simulink library "IOBlock_Library_TTC580"  (R2021a)
settings: Solver=ode45  StartTime=0.0  StopTime=10.0  RelTol=1e-3
PreLoadFcn:
  | addpath(genpath(fileparts(which('IOBlock_Library_TTC580'))));
  | %addpath(genpath(fileparts(which('IOBlock_Library_TTC580.mdl'))))
  | try
  | addpath(genpath([fileparts(which('IOBlock_Library_TTC580')),'\..\DBC_Importer']));
  | addpath(genpath([fileparts(which('IOBlock_Library_TTC580')),'\..\EEPROM_Importer']));
  | addpath(genpath([fileparts(which('IOBlock_Library_TTC580')),'\..\UserDoc']));
  | catch
  | warning('IOBlock_Library_TTC580: add path to DBC_Importer and EEPROM_Importer manually');
  | end
  | try
  | if exist('..\CustomPackage\scripts\OpenAllPackages.m','file')
  |      run('..\CustomPackage\scripts\OpenAllPackages.m'); %always available, ggf. empty
  | end
  | catch
  | warning('A problem occurred opening automatically the CustomPackage. Please open libraries manually');
  | end
  | try
  | set_param(0,'EditorSmartEditingHotParam','off');
  | catch
  | warning('Simlink preferences for ''Edit key parameter when adding new blocks'' needs to be unchecked manually');
  | end
undefined symbols (not defined in the file or in its folder): ADC_Absolute_10V, ADC_Absolute_32V, ADC_Absolute_5V, ADC_BoardTemp, ADC_ChannelInit, ADC_Current, ADC_Get, ADC_K15_, ADC_Ratiometric_10V, ADC_Ratiometric_5V, ADC_Resistive, ADC_SensorSupply, ADC_UBAT, bit_packing, bit_unpacking, CAN_ConfigMsg, compare2error, compare2FET_PROT_REENABLE, crc32_calc_intern, CRC32_EEPROM_Read, CRC32_EEPROM_Write, DIAG_EnterSafestate, DIAG_Status, DIAG_Status_internal, EEPROM_Mirror, EEPROM_Read, EEPROM_Read_OffsetIn, EEPROM_Read_Raw, EEPROM_Write, EEPROM_Write_OffsetIn, EEPROM_Write_Raw, EnterSafestate, FPU_Handler, Get_DI, Get_DI_VarThreshold, Get_K15_, Get_Pulse_Freq_Curr, Get_Pulse_Freq_Volt, Get_WakeUp, GetDateAndTime, IO_ADC_ResetProtection, IO_Blk_Lib_TTC500, IO_CAN_ReadMsg, IO_CAN_WriteMsg, IO_DI_Get, IO_DI_Init, IO_DI_Init_Var, IO_DO_GetCur, IO_DO_GetVoltage, IO_DO_Init, IO_DO_ResetProtection, IO_DO_Set, IO_Driver_GetSerialNumber, IO_Driver_GetVersionOfDriver, IO_Driver_GetVersionOfFPGA, IO_EEPROM_GetStatus, IO_EEPROM_Init, IO_EEPROM_Read_raw, IO_EEPROM_Write, IO_EEPROM_Write_OffsetIn ... (+73)
libraries: simulink x43
(part 15 of 18)

== system IOBlock_Library_TTC580/System  Blocks TTC580 IOlib/Power_Enable ==
  enable : Inport  OutDataTypeStr=boolean  PortDimensions=1
  Data Type Conversion : DataTypeConversion  OutDataTypeStr=uint8
  IO_POWER_Set_POWERSTAGE : Subsystem  LoadFcn=|  mask(IO_POWER_Set_Code){SampleTime=-1, ttlib=IO_Blk_Lib_TTC500, ttDescription=IO_POWER_Set, tt_iolib_version=0.19, pin=IO_INT_POWERSTAGE_ENABLE}
      | try
      | %
      | %Upgrade Information - standard BEGIN
      | new_color = 'blue';
      | new_ver = '0.19';
      | act_ver = get_param(gcb,'tt_iolib_version');
      | if not(strcmp(act_ver,new_ver))
      |     disp(['Upgrade block: ',gcb,char(10),'       Version: ',act_ver,' -> ',new_ver]);
      |     %switch - case for specific upgrade information e.g. additional parameter required 
      |     %Change appearance and version information
      |     set_param(gcb,'ForegroundColor',new_color);
      |     set_param(gcb,'tt_iolib_version',new_ver);
      | end
      | %Upgrade Information - standard END
      | catch
      | %Standard catch section BEGIN 
      | disp(' ');
      | disp('------------------------------------------------------------');
      | disp('An error occurred in a callback of the TTC580-BlockLib.');
      | disp(['Please check the parameters in the mask of ',gcb]);
      | disp('If you do not encounter any violations, then please '); 
      | disp('copy the following lines and report this to support@ttcontrol.com ');
      | disp('<< begin of error message dump >>');
      | disp(['Version of TTC580-BlockLib: ', get_param(gcb,'tt_iolib_version')]);
      | disp(get_param(gcb,'ttDescription'));
      | disp(gcb);
      | x=lasterror;disp(x.message);
      | disp(get_param(gcb,'MaskValues'));
      | disp(version);
      | disp(computer);
      | disp('<< end of error message dump >>');
      | disp('------------------------------------------------------------');
      | disp(' ');
      | %Standard catch section END
      | end
      mask help: Sets a certain mode of the Power IC.
      mask init:
      | %
      settings: CopyFcn=%deleted
      mask Help: web(which('IO_POWER.h'))
      mask TypeOptions pin: IO_INT_POWERSTAGE_ENABLE | IO_SENSOR_SUPPLY_0 | IO_SENSOR_SUPPLY_1 | IO_SENSOR_SUPPLY_2 | IO_INT_SAFETY_SW_0 | IO_INT_SAFETY_SW_1 | IO_INT_SAFETY_SW_2 | IO_K15 | IO_WAKEUP
      mask Callback pin: %
  IO_POWER_Set_SSW0 : Subsystem  LoadFcn=|  mask(IO_POWER_Set_Code){SampleTime=-1, ttlib=IO_Blk_Lib_TTC500, ttDescription=IO_POWER_Set, tt_iolib_version=0.19, pin=IO_INT_SAFETY_SW_0}
      | try
      | %
      | %Upgrade Information - standard BEGIN
      | new_color = 'blue';
      | new_ver = '0.19';
      | act_ver = get_param(gcb,'tt_iolib_version');
      | if not(strcmp(act_ver,new_ver))
      |     disp(['Upgrade block: ',gcb,char(10),'       Version: ',act_ver,' -> ',new_ver]);
      |     %switch - case for specific upgrade information e.g. additional parameter required 
      |     %Change appearance and version information
      |     set_param(gcb,'ForegroundColor',new_color);
      |     set_param(gcb,'tt_iolib_version',new_ver);
      | end
      | %Upgrade Information - standard END
      | catch
      | %Standard catch section BEGIN 
      | disp(' ');
      | disp('------------------------------------------------------------');
      | disp('An error occurred in a callback of the TTC580-BlockLib.');
      | disp(['Please check the parameters in the mask of ',gcb]);
      | disp('If you do not encounter any violations, then please '); 
      | disp('copy the following lines and report this to support@ttcontrol.com ');
      | disp('<< begin of error message dump >>');
      | disp(['Version of TTC580-BlockLib: ', get_param(gcb,'tt_iolib_version')]);
      | disp(get_param(gcb,'ttDescription'));
      | disp(gcb);
      | x=lasterror;disp(x.message);
      | disp(get_param(gcb,'MaskValues'));
      | disp(version);
      | disp(computer);
      | disp('<< end of error message dump >>');
      | disp('------------------------------------------------------------');
      | disp(' ');
      | %Standard catch section END
      | end
      mask help: Sets a certain mode of the Power IC.
      mask init:
      | %
      settings: CopyFcn=%deleted
      mask Help: web(which('IO_POWER.h'))
      mask TypeOptions pin: IO_INT_POWERSTAGE_ENABLE | IO_SENSOR_SUPPLY_0 | IO_SENSOR_SUPPLY_1 | IO_SENSOR_SUPPLY_2 | IO_INT_SAFETY_SW_0 | IO_INT_SAFETY_SW_1 | IO_INT_SAFETY_SW_2 | IO_K15 | IO_WAKEUP
      mask Callback pin: %
  IO_POWER_Set_SSW1 : Subsystem  LoadFcn=|  mask(IO_POWER_Set_Code){SampleTime=-1, ttlib=IO_Blk_Lib_TTC500, ttDescription=IO_POWER_Set, tt_iolib_version=0.19, pin=IO_INT_SAFETY_SW_1}
      | try
      | %
      | %Upgrade Information - standard BEGIN
      | new_color = 'blue';
      | new_ver = '0.19';
      | act_ver = get_param(gcb,'tt_iolib_version');
      | if not(strcmp(act_ver,new_ver))
      |     disp(['Upgrade block: ',gcb,char(10),'       Version: ',act_ver,' -> ',new_ver]);
      |     %switch - case for specific upgrade information e.g. additional parameter required 
      |     %Change appearance and version information
      |     set_param(gcb,'ForegroundColor',new_color);
      |     set_param(gcb,'tt_iolib_version',new_ver);
      | end
      | %Upgrade Information - standard END
      | catch
      | %Standard catch section BEGIN 
      | disp(' ');
      | disp('------------------------------------------------------------');
      | disp('An error occurred in a callback of the TTC580-BlockLib.');
      | disp(['Please check the parameters in the mask of ',gcb]);
      | disp('If you do not encounter any violations, then please '); 
      | disp('copy the following lines and report this to support@ttcontrol.com ');
      | disp('<< begin of error message dump >>');
      | disp(['Version of TTC580-BlockLib: ', get_param(gcb,'tt_iolib_version')]);
      | disp(get_param(gcb,'ttDescription'));
      | disp(gcb);
      | x=lasterror;disp(x.message);
      | disp(get_param(gcb,'MaskValues'));
      | disp(version);
      | disp(computer);
      | disp('<< end of error message dump >>');
      | disp('------------------------------------------------------------');
      | disp(' ');
      | %Standard catch section END
      | end
      mask help: Sets a certain mode of the Power IC.
      mask init:
      | %
      settings: CopyFcn=%deleted
      mask Help: web(which('IO_POWER.h'))
      mask TypeOptions pin: IO_INT_POWERSTAGE_ENABLE | IO_SENSOR_SUPPLY_0 | IO_SENSOR_SUPPLY_1 | IO_SENSOR_SUPPLY_2 | IO_INT_SAFETY_SW_0 | IO_INT_SAFETY_SW_1 | IO_INT_SAFETY_SW_2 | IO_K15 | IO_WAKEUP
      mask Callback pin: %
  IO_POWER_Set_SSW2 : Subsystem  LoadFcn=|  mask(IO_POWER_Set_Code){SampleTime=-1, ttlib=IO_Blk_Lib_TTC500, ttDescription=IO_POWER_Set, tt_iolib_version=0.19, pin=IO_INT_SAFETY_SW_2}
      | try
      | %
      | %Upgrade Information - standard BEGIN
      | new_color = 'blue';
      | new_ver = '0.19';
      | act_ver = get_param(gcb,'tt_iolib_version');
      | if not(strcmp(act_ver,new_ver))
      |     disp(['Upgrade block: ',gcb,char(10),'       Version: ',act_ver,' -> ',new_ver]);
      |     %switch - case for specific upgrade information e.g. additional parameter required 
      |     %Change appearance and version information
      |     set_param(gcb,'ForegroundColor',new_color);
      |     set_param(gcb,'tt_iolib_version',new_ver);
      | end
      | %Upgrade Information - standard END
      | catch
      | %Standard catch section BEGIN 
      | disp(' ');
      | disp('------------------------------------------------------------');
      | disp('An error occurred in a callback of the TTC580-BlockLib.');
      | disp(['Please check the parameters in the mask of ',gcb]);
      | disp('If you do not encounter any violations, then please '); 
      | disp('copy the following lines and report this to support@ttcontrol.com ');
      | disp('<< begin of error message dump >>');
      | disp(['Version of TTC580-BlockLib: ', get_param(gcb,'tt_iolib_version')]);
      | disp(get_param(gcb,'ttDescription'));
      | disp(gcb);
      | x=lasterror;disp(x.message);
      | disp(get_param(gcb,'MaskValues'));
      | disp(version);
      | disp(computer);
      | disp('<< end of error message dump >>');
      | disp('------------------------------------------------------------');
      | disp(' ');
      | %Standard catch section END
      | end
      mask help: Sets a certain mode of the Power IC.
      mask init:
      | %
      settings: CopyFcn=%deleted
      mask Help: web(which('IO_POWER.h'))
      mask TypeOptions pin: IO_INT_POWERSTAGE_ENABLE | IO_SENSOR_SUPPLY_0 | IO_SENSOR_SUPPLY_1 | IO_SENSOR_SUPPLY_2 | IO_INT_SAFETY_SW_0 | IO_INT_SAFETY_SW_1 | IO_INT_SAFETY_SW_2 | IO_K15 | IO_WAKEUP
      mask Callback pin: %
  Terminator_enable{,1..3} (4 alike) : Terminator
  wires:
  enable/1 -> Data Type Conversion/1
  Data Type Conversion/1 -> IO_POWER_Set_POWERSTAGE/1(mode), IO_POWER_Set_SSW0/1(mode), IO_POWER_Set_SSW1/1(mode), IO_POWER_Set_SSW2/1(mode)
  IO_POWER_Set_POWERSTAGE/1(ErrorCode) -> Terminator_enable/1
  IO_POWER_Set_SSW0/1(ErrorCode) -> Terminator_enable1/1
  IO_POWER_Set_SSW1/1(ErrorCode) -> Terminator_enable2/1
  IO_POWER_Set_SSW2/1(ErrorCode) -> Terminator_enable3/1

== system IOBlock_Library_TTC580/System  Blocks TTC580 IOlib/SetDateAndTime ==
  trigger : Inport  OutDataTypeStr=boolean  PortDimensions=1
  seconds : Inport  Port=2  OutDataTypeStr=uint8  PortDimensions=1
  minutes : Inport  Port=3  OutDataTypeStr=uint8  PortDimensions=1
  hours : Inport  Port=4  OutDataTypeStr=uint8  PortDimensions=1
  days : Inport  Port=5  OutDataTypeStr=uint8  PortDimensions=1
  months : Inport  Port=6  OutDataTypeStr=uint8  PortDimensions=1
  years : Inport  Port=7  OutDataTypeStr=uint8  PortDimensions=1
  IO_RTC_GetDateAndTimeStatus : Subsystem  LoadFcn=|  mask(IO_RTC_GetDateAndTimeStatus_Code){SampleTime=-1, ttlib=IO_Blk_Lib_TTC500, ttDescription=IO_RTC_GetDateAndTimeStatus, tt_iolib_version=0.19}
      | try
      | %
      | %Upgrade Information - standard BEGIN
      | new_color = 'blue';
      | new_ver = '0.19';
      | act_ver = get_param(gcb,'tt_iolib_version');
      | if not(strcmp(act_ver,new_ver))
      |     disp(['Upgrade block: ',gcb,char(10),'       Version: ',act_ver,' -> ',new_ver]);
      |     %switch - case for specific upgrade information e.g. additional parameter required 
      |     %Change appearance and version information
      |     set_param(gcb,'ForegroundColor',new_color);
      |     set_param(gcb,'tt_iolib_version',new_ver);
      | end
      | %Upgrade Information - standard END
      | catch
      | %Standard catch section BEGIN 
      | disp(' ');
      | disp('------------------------------------------------------------');
      | disp('An error occurred in a callback of the TTC580-BlockLib.');
      | disp(['Please check the parameters in the mask of ',gcb]);
      | disp('If you do not encounter any violations, then please '); 
      | disp('copy the following lines and report this to support@ttcontrol.com ');
      | disp('<< begin of error message dump >>');
      | disp(['Version of TTC580-BlockLib: ', get_param(gcb,'tt_iolib_version')]);
      | disp(get_param(gcb,'ttDescription'));
      | disp(gcb);
      | x=lasterror;disp(x.message);
      | disp(get_param(gcb,'MaskValues'));
      | disp(version);
      | disp(computer);
      | disp('<< end of error message dump >>');
      | disp('------------------------------------------------------------');
      | disp(' ');
      | %Standard catch section END
      | end
      mask help: Gets the status of the external RTC device.
      mask init:
      | %
      settings: CopyFcn=%deleted
      mask Help: No further help available for this block
  IO_RTC_InitDateAndTime : Subsystem  LoadFcn=|  mask(IO_RTC_InitDateAndTime_Code){SampleTime=-1, ttlib=IO_Blk_Lib_TTC500, ttDescription=IO_RTC_InitDateAndTime, tt_iolib_version=0.19}
      | try
      | %
      | %Upgrade Information - standard BEGIN
      | new_color = 'blue';
      | new_ver = '0.19';
      | act_ver = get_param(gcb,'tt_iolib_version');
      | if not(strcmp(act_ver,new_ver))
      |     disp(['Upgrade block: ',gcb,char(10),'       Version: ',act_ver,' -> ',new_ver]);
      |     %switch - case for specific upgrade information e.g. additional parameter required 
      |     %Change appearance and version information
      |     set_param(gcb,'ForegroundColor',new_color);
      |     set_param(gcb,'tt_iolib_version',new_ver);
      | end
      | %Upgrade Information - standard END
      | catch
      | %Standard catch section BEGIN 
      | disp(' ');
      | disp('------------------------------------------------------------');
      | disp('An error occurred in a callback of the TTC580-BlockLib.');
      | disp(['Please check the parameters in the mask of ',gcb]);
      | disp('If you do not encounter any violations, then please '); 
      | disp('copy the following lines and report this to support@ttcontrol.com ');
      | disp('<< begin of error message dump >>');
      | disp(['Version of TTC580-BlockLib: ', get_param(gcb,'tt_iolib_version')]);
      | disp(get_param(gcb,'ttDescription'));
      | disp(gcb);
      | x=lasterror;disp(x.message);
      | disp(get_param(gcb,'MaskValues'));
      | disp(version);
      | disp(computer);
      | disp('<< end of error message dump >>');
      | disp('------------------------------------------------------------');
      | disp(' ');
      | %Standard catch section END
      | end
      mask help: Initializes the external RTC device for date and time operations.
      mask init:
      | %
      settings: CopyFcn=%deleted
      mask Help: No further help available for this block
  IO_RTC_SetDateAndTime : Subsystem  LoadFcn=|  mask(IO_RTC_SetDateAndTime_Code){SampleTime=-1, ttlib=IO_Blk_Lib_TTC500, ttDescription=IO_RTC_SetDateAndTime, tt_iolib_version=0.19}
      | try
      | %
      | %Upgrade Information - standard BEGIN
      | new_color = 'blue';
      | new_ver = '0.19';
      | act_ver = get_param(gcb,'tt_iolib_version');
      | if not(strcmp(act_ver,new_ver))
      |     disp(['Upgrade block: ',gcb,char(10),'       Version: ',act_ver,' -> ',new_ver]);
      |     %switch - case for specific upgrade information e.g. additional parameter required 
      |     %Change appearance and version information
      |     set_param(gcb,'ForegroundColor',new_color);
      |     set_param(gcb,'tt_iolib_version',new_ver);
      | end
      | %Upgrade Information - standard END
      | catch
      | %Standard catch section BEGIN 
      | disp(' ');
      | disp('------------------------------------------------------------');
      | disp('An error occurred in a callback of the TTC580-BlockLib.');
      | disp(['Please check the parameters in the mask of ',gcb]);
      | disp('If you do not encounter any violations, then please '); 
      | disp('copy the following lines and report this to support@ttcontrol.com ');
      | disp('<< begin of error message dump >>');
      | disp(['Version of TTC580-BlockLib: ', get_param(gcb,'tt_iolib_version')]);
      | disp(get_param(gcb,'ttDescription'));
      | disp(gcb);
      | x=lasterror;disp(x.message);
      | disp(get_param(gcb,'MaskValues'));
      | disp(version);
      | disp(computer);
      | disp('<< end of error message dump >>');
      | disp('------------------------------------------------------------');
      | disp(' ');
      | %Standard catch section END
      | end
      mask help: Sets the date and time of the real time clock.
      mask init:
      | %
      settings: CopyFcn=%deleted
      mask Help: No further help available for this block
  Terminator : Terminator
  Status : Outport  VectorParamsAs1DForOutWhenUnconnected=off
  wires:
  years/1 -> IO_RTC_SetDateAndTime/6(years)
  months/1 -> IO_RTC_SetDateAndTime/5(months)
  days/1 -> IO_RTC_SetDateAndTime/4(days)
  hours/1 -> IO_RTC_SetDateAndTime/3(hours)
  minutes/1 -> IO_RTC_SetDateAndTime/2(minutes)
  seconds/1 -> IO_RTC_SetDateAndTime/1(seconds)
  trigger/1 -> IO_RTC_SetDateAndTime/Trigger
  IO_RTC_SetDateAndTime/1(ErrorCode) -> IO_RTC_GetDateAndTimeStatus/1(logical_link)
  IO_RTC_GetDateAndTimeStatus/1(ErrorCode) -> Status/1
  IO_RTC_InitDateAndTime/1(ErrorCode) -> Terminator/1

== system IOBlock_Library_TTC580/System  Blocks TTC580 IOlib/compare2error ==
  Errorcode : Inport
  compare2error_s : S-Function  FunctionName=compare2error_s  Parameters=SampleTime,define  SFunctionDeploymentMode=off  EnableBusSupport=off
  b_compare : Outport  VectorParamsAs1DForOutWhenUnconnected=off
  wires:
  compare2error_s/1 -> b_compare/1
  Errorcode/1 -> compare2error_s/1

== system IOBlock_Library_TTC580/UART TTC580 IOlib/UART_Read ==
  Constant : Constant  Value=size_of_data  OutDataTypeStr=uint16
  IO_UART_Init : Subsystem  LoadFcn=|  mask(IO_UART_Init_Code){SampleTime=-1, ttlib=IO_Blk_Lib_TTC500, ttDescription=IO_UART_Init, tt_iolib_version=0.25, baudrate=baudrate, dbits=dbits, par=par, sbits=sbits}
      | try
      | %
      | %Upgrade Information - standard BEGIN
      | new_color = 'blue';
      | new_ver = '0.25';
      | act_ver = get_param(gcb,'tt_iolib_version');
      | if not(strcmp(act_ver,new_ver))
      |     disp(['Upgrade block: ',gcb,char(10),'       Version: ',act_ver,' to ',new_ver]);
      |     %switch - case for specific upgrade information e.g. additional parameter required 
      |     %Change appearance and version information
      |     set_param(gcb,'ForegroundColor',new_color);
      |     set_param(gcb,'tt_iolib_version',new_ver);
      | end
      | %Upgrade Information - standard END
      | catch
      | %Standard catch section BEGIN
      | errordlg('An error occurred in a callback of the TTC580-BlockLib. Please open the Diagnostic Viewer for further details');
      | disp(' ');
      | disp('------------------------------------------------------------');
      | disp('An error occurred in a callback of the TTC580-BlockLib.');
      | disp(['Please check the parameters in the mask of ',gcb]);
      | disp('If you do not encounter any violations, then please '); 
      | disp('copy the following lines and report this to support@ttcontrol.com ');
      | disp('<< begin of error message dump >>');
      | disp(['Version of TTC580-BlockLib: ', get_param(gcb,'tt_iolib_version')]);
      | disp(get_param(gcb,'ttDescription'));
      | disp(gcb);
      | x=lasterror;disp(x.message);
      | disp(get_param(gcb,'MaskValues'));
      | disp(version);
      | disp(computer);
      | disp('<< end of error message dump >>');
      | disp('------------------------------------------------------------');
      | disp(' ');
      | %Standard catch section END
      | end
      mask help: Initialization of the UART communication driver.
      mask init:
      | %
      settings: CopyFcn=%deleted
      mask Help: No further help available for this block
      mask Callback baudrate: %
      mask Callback dbits: %
      mask Callback par: %
      mask Callback sbits: %
  IO_UART_Read : Subsystem  LoadFcn=|  mask(IO_UART_Read_Code){SampleTime=-1, ttlib=IO_Blk_Lib_TTC500, ttDescription=IO_UART_Read, tt_iolib_version=0.25}
      | try
      | %
      | %Upgrade Information - standard BEGIN
      | new_color = 'blue';
      | new_ver = '0.25';
      | act_ver = get_param(gcb,'tt_iolib_version');
      | if not(strcmp(act_ver,new_ver))
      |     disp(['Upgrade block: ',gcb,char(10),'       Version: ',act_ver,' to ',new_ver]);
      |     %switch - case for specific upgrade information e.g. additional parameter required 
      |     %Change appearance and version information
      |     set_param(gcb,'ForegroundColor',new_color);
      |     set_param(gcb,'tt_iolib_version',new_ver);
      | end
      | %Upgrade Information - standard END
      | catch
      | %Standard catch section BEGIN
      | errordlg('An error occurred in a callback of the TTC580-BlockLib. Please open the Diagnostic Viewer for further details');
      | disp(' ');
      | disp('------------------------------------------------------------');
      | disp('An error occurred in a callback of the TTC580-BlockLib.');
      | disp(['Please check the parameters in the mask of ',gcb]);
      | disp('If you do not encounter any violations, then please '); 
      | disp('copy the following lines and report this to support@ttcontrol.com ');
      | disp('<< begin of error message dump >>');
      | disp(['Version of TTC580-BlockLib: ', get_param(gcb,'tt_iolib_version')]);
      | disp(get_param(gcb,'ttDescription'));
      | disp(gcb);
      | x=lasterror;disp(x.message);
      | disp(get_param(gcb,'MaskValues'));
      | disp(version);
      | disp(computer);
      | disp('<< end of error message dump >>');
      | disp('------------------------------------------------------------');
      | disp(' ');
      | %Standard catch section END
      | end
      mask help: Read data from serial interface.
      mask init:
      | %
      settings: CopyFcn=%deleted
      mask Help: No further help available for this block
  Terminator_value2 : Terminator
  ErrorCode : Outport  VectorParamsAs1DForOutWhenUnconnected=off
  data : Outport  Port=2  PortDimensions=size_of_data  VectorParamsAs1DForOutWhenUnconnected=off
  rx_len : Outport  Port=3  VectorParamsAs1DForOutWhenUnconnected=off
  wires:
  IO_UART_Read/3(rx_len) -> rx_len/1
  IO_UART_Read/2(data) -> data/1
  IO_UART_Read/1(ErrorCode) -> ErrorCode/1
  Constant/1 -> IO_UART_Read/1(len)
  IO_UART_Init/1(ErrorCode) -> Terminator_value2/1

== system IOBlock_Library_TTC580/UART TTC580 IOlib/UART_Write ==
  value : Inport
  Constant : Constant  Value=0  OutDataTypeStr=uint16
  Data Type Conversion : DataTypeConversion  OutDataTypeStr=uint16
  IO_UART_Init : Subsystem  LoadFcn=|  mask(IO_UART_Init_Code){SampleTime=-1, ttlib=IO_Blk_Lib_TTC500, ttDescription=IO_UART_Init, tt_iolib_version=0.25, baudrate=baudrate, dbits=dbits, par=par, sbits=sbits}
      | try
      | %
      | %Upgrade Information - standard BEGIN
      | new_color = 'blue';
      | new_ver = '0.25';
      | act_ver = get_param(gcb,'tt_iolib_version');
      | if not(strcmp(act_ver,new_ver))
      |     disp(['Upgrade block: ',gcb,char(10),'       Version: ',act_ver,' to ',new_ver]);
      |     %switch - case for specific upgrade information e.g. additional parameter required 
      |     %Change appearance and version information
      |     set_param(gcb,'ForegroundColor',new_color);
      |     set_param(gcb,'tt_iolib_version',new_ver);
      | end
      | %Upgrade Information - standard END
      | catch
      | %Standard catch section BEGIN
      | errordlg('An error occurred in a callback of the TTC580-BlockLib. Please open the Diagnostic Viewer for further details');
      | disp(' ');
      | disp('------------------------------------------------------------');
      | disp('An error occurred in a callback of the TTC580-BlockLib.');
      | disp(['Please check the parameters in the mask of ',gcb]);
      | disp('If you do not encounter any violations, then please '); 
      | disp('copy the following lines and report this to support@ttcontrol.com ');
      | disp('<< begin of error message dump >>');
      | disp(['Version of TTC580-BlockLib: ', get_param(gcb,'tt_iolib_version')]);
      | disp(get_param(gcb,'ttDescription'));
      | disp(gcb);
      | x=lasterror;disp(x.message);
      | disp(get_param(gcb,'MaskValues'));
      | disp(version);
      | disp(computer);
      | disp('<< end of error message dump >>');
      | disp('------------------------------------------------------------');
      | disp(' ');
      | %Standard catch section END
      | end
      mask help: Initialization of the UART communication driver.
      mask init:
      | %
      settings: CopyFcn=%deleted
      mask Help: No further help available for this block
      mask Callback baudrate: %
      mask Callback dbits: %
      mask Callback par: %
      mask Callback sbits: %
  IO_UART_Write : Subsystem  LoadFcn=|  mask(IO_UART_Write_Code){SampleTime=-1, ttlib=IO_Blk_Lib_TTC500, ttDescription=IO_UART_Write, tt_iolib_version=0.25}
      | try
      | %
      | %Upgrade Information - standard BEGIN
      | new_color = 'blue';
      | new_ver = '0.25';
      | act_ver = get_param(gcb,'tt_iolib_version');
      | if not(strcmp(act_ver,new_ver))
      |     disp(['Upgrade block: ',gcb,char(10),'       Version: ',act_ver,' to ',new_ver]);
      |     %switch - case for specific upgrade information e.g. additional parameter required 
      |     %Change appearance and version information
      |     set_param(gcb,'ForegroundColor',new_color);
      |     set_param(gcb,'tt_iolib_version',new_ver);
      | end
      | %Upgrade Information - standard END
      | catch
      | %Standard catch section BEGIN
      | errordlg('An error occurred in a callback of the TTC580-BlockLib. Please open the Diagnostic Viewer for further details');
      | disp(' ');
      | disp('------------------------------------------------------------');
      | disp('An error occurred in a callback of the TTC580-BlockLib.');
      | disp(['Please check the parameters in the mask of ',gcb]);
      | disp('If you do not encounter any violations, then please '); 
      | disp('copy the following lines and report this to support@ttcontrol.com ');
      | disp('<< begin of error message dump >>');
      | disp(['Version of TTC580-BlockLib: ', get_param(gcb,'tt_iolib_version')]);
      | disp(get_param(gcb,'ttDescription'));
      | disp(gcb);
      | x=lasterror;disp(x.message);
      | disp(get_param(gcb,'MaskValues'));
      | disp(version);
      | disp(computer);
      | disp('<< end of error message dump >>');
      | disp('------------------------------------------------------------');
      | disp(' ');
      | %Standard catch section END
      | end
      mask help: Write data to serial interface.
      mask init:
      | %
      settings: CopyFcn=%deleted  RTWSystemCode=Inline
      mask Help: No further help available for this block
  Saturation Dynamic : simulink/Discontinuities/Saturation Dynamic  OutMin=[]  OutMax=[]  OutDataTypeStr=uint16  OutputDataTypeScalingMode=uint16  OutDataType=fixdt(1, 16)  OutScaling=2^-10  DoSatur=off
  Terminator2 : Terminator
  Terminator_value2 : Terminator
  Trigger : Subsystem  mask(Derate Trigger){derate=derate_val}
      mask help: derate "n": every n-th cylce a trigger is submitted
  Width : Width  DataType=uint16
  snprintf : Subsystem  LoadFcn=|  mask(snprintf_Code){SampleTime=-1, ttlib=IO_Blk_Lib_TTC500, ttDescription=snprintf, tt_iolib_version=0.25, max_size=max_size, Comment=Comment}
      | try
      | %
      | %Upgrade Information - standard BEGIN
      | new_color = 'blue';
      | new_ver = '0.25';
      | act_ver = get_param(gcb,'tt_iolib_version');
      | if not(strcmp(act_ver,new_ver))
      |     disp(['Upgrade block: ',gcb,char(10),'       Version: ',act_ver,' to ',new_ver]);
      |     %switch - case for specific upgrade information e.g. additional parameter required 
      |     %Change appearance and version information
      |     set_param(gcb,'ForegroundColor',new_color);
      |     set_param(gcb,'tt_iolib_version',new_ver);
      | end
      | %Upgrade Information - standard END
      | catch
      | %Standard catch section BEGIN
      | errordlg('An error occurred in a callback of the TTC580-BlockLib. Please open the Diagnostic Viewer for further details');
      | disp(' ');
      | disp('------------------------------------------------------------');
      | disp('An error occurred in a callback of the TTC580-BlockLib.');
      | disp(['Please check the parameters in the mask of ',gcb]);
      | disp('If you do not encounter any violations, then please '); 
      | disp('copy the following lines and report this to support@ttcontrol.com ');
      | disp('<< begin of error message dump >>');
      | disp(['Version of TTC580-BlockLib: ', get_param(gcb,'tt_iolib_version')]);
      | disp(get_param(gcb,'ttDescription'));
      | disp(gcb);
      | x=lasterror;disp(x.message);
      | disp(get_param(gcb,'MaskValues'));
      | disp(version);
      | disp(computer);
      | disp('<< end of error message dump >>');
      | disp('------------------------------------------------------------');
      | disp(' ');
      | %Standard catch section END
      | end
      mask help: The C library function snprintf sends formatted output to a string with maximum length of n characters.
      mask init:
      | %
      settings: CopyFcn=%deleted
      mask Help: No further help available for this block
      mask Callback max_size: %
      mask Callback Comment: %
  ErrorCode : Outport  VectorParamsAs1DForOutWhenUnconnected=off
  wires:
  IO_UART_Write/2(tx_len) -> Terminator2/1
  Constant/1 -> Saturation Dynamic/3
  Width/1 -> Saturation Dynamic/1
  Saturation Dynamic/1 -> IO_UART_Write/2(len)
  Trigger/1(Trigger) -> IO_UART_Write/Enable
  snprintf/1(NumOfChar) -> Data Type Conversion/1
  Data Type Conversion/1 -> Saturation Dynamic/2
  IO_UART_Init/1(ErrorCode) -> Terminator_value2/1
  IO_UART_Write/1(ErrorCode) -> ErrorCode/1
  value/1 -> snprintf/1(value)
  snprintf/2(str_out) -> IO_UART_Write/1(data), Width/1

== system IOBlock_Library_TTC580/UART TTC580 IOlib/Write_RS232_ ==
  value : Inport
  Constant : Constant  Value=0  OutDataTypeStr=uint16
  Data Type Conversion : DataTypeConversion  OutDataTypeStr=uint16
  IO_UART_Init : Subsystem  LoadFcn=|  mask(IO_UART_Init_Code){SampleTime=-1, ttlib=IO_Blk_Lib_TTC500, ttDescription=IO_UART_Init, tt_iolib_version=0.25, baudrate=115200, dbits='8', par='IO_UART_PARITY_NONE', sbits='1'}
      | try
      | %
      | %Upgrade Information - standard BEGIN
      | new_color = 'blue';
      | new_ver = '0.25';
      | act_ver = get_param(gcb,'tt_iolib_version');
      | if not(strcmp(act_ver,new_ver))
      |     disp(['Upgrade block: ',gcb,char(10),'       Version: ',act_ver,' to ',new_ver]);
      |     %switch - case for specific upgrade information e.g. additional parameter required 
      |     %Change appearance and version information
      |     set_param(gcb,'ForegroundColor',new_color);
      |     set_param(gcb,'tt_iolib_version',new_ver);
      | end
      | %Upgrade Information - standard END
      | catch
      | %Standard catch section BEGIN
      | errordlg('An error occurred in a callback of the TTC580-BlockLib. Please open the Diagnostic Viewer for further details');
      | disp(' ');
      | disp('------------------------------------------------------------');
      | disp('An error occurred in a callback of the TTC580-BlockLib.');
      | disp(['Please check the parameters in the mask of ',gcb]);
      | disp('If you do not encounter any violations, then please '); 
      | disp('copy the following lines and report this to support@ttcontrol.com ');
      | disp('<< begin of error message dump >>');
      | disp(['Version of TTC580-BlockLib: ', get_param(gcb,'tt_iolib_version')]);
      | disp(get_param(gcb,'ttDescription'));
      | disp(gcb);
      | x=lasterror;disp(x.message);
      | disp(get_param(gcb,'MaskValues'));
      | disp(version);
      | disp(computer);
      | disp('<< end of error message dump >>');
      | disp('------------------------------------------------------------');
      | disp(' ');
      | %Standard catch section END
      | end
      mask help: Initialization of the UART communication driver.
      mask init:
      | %
      settings: CopyFcn=%deleted
      mask Help: No further help available for this block
      mask Callback baudrate: %
      mask Callback dbits: %
      mask Callback par: %
      mask Callback sbits: %
  IO_UART_Write : Subsystem  LoadFcn=|  mask(IO_UART_Write_Code){SampleTime=-1, ttlib=IO_Blk_Lib_TTC500, ttDescription=IO_UART_Write, tt_iolib_version=0.25}
      | try
      | %
      | %Upgrade Information - standard BEGIN
      | new_color = 'blue';
      | new_ver = '0.25';
      | act_ver = get_param(gcb,'tt_iolib_version');
      | if not(strcmp(act_ver,new_ver))
      |     disp(['Upgrade block: ',gcb,char(10),'       Version: ',act_ver,' to ',new_ver]);
      |     %switch - case for specific upgrade information e.g. additional parameter required 
      |     %Change appearance and version information
      |     set_param(gcb,'ForegroundColor',new_color);
      |     set_param(gcb,'tt_iolib_version',new_ver);
      | end
      | %Upgrade Information - standard END
      | catch
      | %Standard catch section BEGIN
      | errordlg('An error occurred in a callback of the TTC580-BlockLib. Please open the Diagnostic Viewer for further details');
      | disp(' ');
      | disp('------------------------------------------------------------');
      | disp('An error occurred in a callback of the TTC580-BlockLib.');
      | disp(['Please check the parameters in the mask of ',gcb]);
      | disp('If you do not encounter any violations, then please '); 
      | disp('copy the following lines and report this to support@ttcontrol.com ');
      | disp('<< begin of error message dump >>');
      | disp(['Version of TTC580-BlockLib: ', get_param(gcb,'tt_iolib_version')]);
      | disp(get_param(gcb,'ttDescription'));
      | disp(gcb);
      | x=lasterror;disp(x.message);
      | disp(get_param(gcb,'MaskValues'));
      | disp(version);
      | disp(computer);
      | disp('<< end of error message dump >>');
      | disp('------------------------------------------------------------');
      | disp(' ');
      | %Standard catch section END
      | end
      mask help: Write data to serial interface.
      mask init:
      | %
      settings: CopyFcn=%deleted  RTWSystemCode=Inline
      mask Help: No further help available for this block
  Saturation Dynamic : simulink/Discontinuities/Saturation Dynamic  OutMin=[]  OutMax=[]  OutDataTypeStr=uint16  OutputDataTypeScalingMode=uint16  OutDataType=fixdt(1, 16)  OutScaling=2^-10  DoSatur=off
  Terminator2 : Terminator
  Terminator_value1 : Terminator
  Terminator_value2 : Terminator
  Trigger : Subsystem  mask(Derate Trigger){derate=derate_val}
      mask help: derate "n": every n-th cylce a trigger is submitted
  Width : Width  DataType=uint16
  snprintf_merge_printf : Subsystem  LoadFcn=|  mask(snprintf_merge_printf_Code){SampleTime=-1, ttlib=IO_Blk_Lib_TTC500, ttDescription=snprintf_merge_printf, tt_iolib_version=0.25, max_size=80, Comment=Comment}
      | try
      | %
      | %Upgrade Information - standard BEGIN
      | new_color = 'blue';
      | new_ver = '0.25';
      | act_ver = get_param(gcb,'tt_iolib_version');
      | if not(strcmp(act_ver,new_ver))
      |     disp(['Upgrade block: ',gcb,char(10),'       Version: ',act_ver,' to ',new_ver]);
      |     %switch - case for specific upgrade information e.g. additional parameter required 
      |     %Change appearance and version information
      |     set_param(gcb,'ForegroundColor',new_color);
      |     set_param(gcb,'tt_iolib_version',new_ver);
      | end
      | %Upgrade Information - standard END
      | catch
      | %Standard catch section BEGIN
      | errordlg('An error occurred in a callback of the TTC580-BlockLib. Please open the Diagnostic Viewer for further details');
      | disp(' ');
      | disp('------------------------------------------------------------');
      | disp('An error occurred in a callback of the TTC580-BlockLib.');
      | disp(['Please check the parameters in the mask of ',gcb]);
      | disp('If you do not encounter any violations, then please '); 
      | disp('copy the following lines and report this to support@ttcontrol.com ');
      | disp('<< begin of error message dump >>');
      | disp(['Version of TTC580-BlockLib: ', get_param(gcb,'tt_iolib_version')]);
      | disp(get_param(gcb,'ttDescription'));
      | disp(gcb);
      | x=lasterror;disp(x.message);
      | disp(get_param(gcb,'MaskValues'));
      | disp(version);
      | disp(computer);
      | disp('<< end of error message dump >>');
      | disp('------------------------------------------------------------');
      | disp(' ');
      | %Standard catch section END
      | end
      mask help:
      | The C library function snprintf sends formatted output to a string with maximum length of n characters.
      | This snprintf implementation adds LF and reset cursor information the way that the printf implementation did it before
      mask init:
      | %
      settings: CopyFcn=%deleted
      mask Help: No further help available for this block
      mask Callback max_size: %
      mask Callback Comment: %
  wires:
  Data Type Conversion/1 -> Saturation Dynamic/2
  Trigger/1(Trigger) -> IO_UART_Write/Enable
  IO_UART_Write/1(ErrorCode) -> Terminator_value1/1
  Constant/1 -> Saturation Dynamic/3
  value/1 -> snprintf_merge_printf/1(value)
  snprintf_merge_printf/1(NumOfChar) -> Data Type Conversion/1
  Width/1 -> Saturation Dynamic/1
  IO_UART_Init/1(ErrorCode) -> Terminator_value2/1
  Saturation Dynamic/1 -> IO_UART_Write/2(len)
  snprintf_merge_printf/2(str_out) -> IO_UART_Write/1(data), Width/1
  IO_UART_Write/2(tx_len) -> Terminator2/1

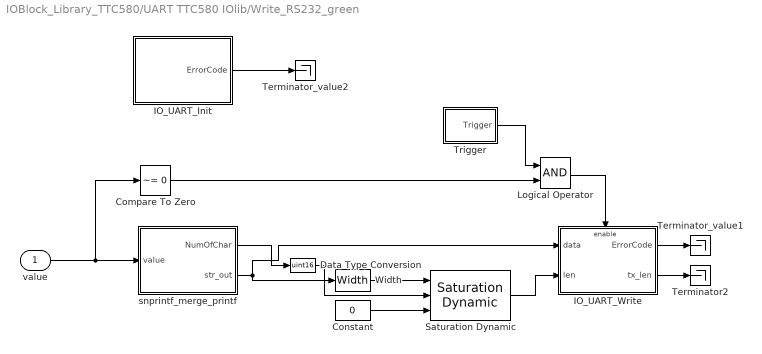
== system IOBlock_Library_TTC580/UART TTC580 IOlib/Write_RS232_green ==
  value : Inport
  Compare To Zero : simulink/Logic and Bit Operations/Compare To Zero  relop=~=  OutDataTypeStr=boolean
  Constant : Constant  Value=0  OutDataTypeStr=uint16
  Data Type Conversion : DataTypeConversion  OutDataTypeStr=uint16
  IO_UART_Init : Subsystem  LoadFcn=|  mask(IO_UART_Init_Code){SampleTime=-1, ttlib=IO_Blk_Lib_TTC500, ttDescription=IO_UART_Init, tt_iolib_version=0.25, baudrate=115200, dbits='8', par='IO_UART_PARITY_NONE', sbits='1'}
      | try
      | %
      | %Upgrade Information - standard BEGIN
      | new_color = 'blue';
      | new_ver = '0.25';
      | act_ver = get_param(gcb,'tt_iolib_version');
      | if not(strcmp(act_ver,new_ver))
      |     disp(['Upgrade block: ',gcb,char(10),'       Version: ',act_ver,' to ',new_ver]);
      |     %switch - case for specific upgrade information e.g. additional parameter required 
      |     %Change appearance and version information
      |     set_param(gcb,'ForegroundColor',new_color);
      |     set_param(gcb,'tt_iolib_version',new_ver);
      | end
      | %Upgrade Information - standard END
      | catch
      | %Standard catch section BEGIN
      | errordlg('An error occurred in a callback of the TTC580-BlockLib. Please open the Diagnostic Viewer for further details');
      | disp(' ');
      | disp('------------------------------------------------------------');
      | disp('An error occurred in a callback of the TTC580-BlockLib.');
      | disp(['Please check the parameters in the mask of ',gcb]);
      | disp('If you do not encounter any violations, then please '); 
      | disp('copy the following lines and report this to support@ttcontrol.com ');
      | disp('<< begin of error message dump >>');
      | disp(['Version of TTC580-BlockLib: ', get_param(gcb,'tt_iolib_version')]);
      | disp(get_param(gcb,'ttDescription'));
      | disp(gcb);
      | x=lasterror;disp(x.message);
      | disp(get_param(gcb,'MaskValues'));
      | disp(version);
      | disp(computer);
      | disp('<< end of error message dump >>');
      | disp('------------------------------------------------------------');
      | disp(' ');
      | %Standard catch section END
      | end
      mask help: Initialization of the UART communication driver.
      mask init:
      | %
      settings: CopyFcn=%deleted
      mask Help: No further help available for this block
      mask Callback baudrate: %
      mask Callback dbits: %
      mask Callback par: %
      mask Callback sbits: %
  IO_UART_Write : Subsystem  LoadFcn=|  mask(IO_UART_Write_Code){SampleTime=-1, ttlib=IO_Blk_Lib_TTC500, ttDescription=IO_UART_Write, tt_iolib_version=0.25}
      | try
      | %
      | %Upgrade Information - standard BEGIN
      | new_color = 'blue';
      | new_ver = '0.25';
      | act_ver = get_param(gcb,'tt_iolib_version');
      | if not(strcmp(act_ver,new_ver))
      |     disp(['Upgrade block: ',gcb,char(10),'       Version: ',act_ver,' to ',new_ver]);
      |     %switch - case for specific upgrade information e.g. additional parameter required 
      |     %Change appearance and version information
      |     set_param(gcb,'ForegroundColor',new_color);
      |     set_param(gcb,'tt_iolib_version',new_ver);
      | end
      | %Upgrade Information - standard END
      | catch
      | %Standard catch section BEGIN
      | errordlg('An error occurred in a callback of the TTC580-BlockLib. Please open the Diagnostic Viewer for further details');
      | disp(' ');
      | disp('------------------------------------------------------------');
      | disp('An error occurred in a callback of the TTC580-BlockLib.');
      | disp(['Please check the parameters in the mask of ',gcb]);
      | disp('If you do not encounter any violations, then please '); 
      | disp('copy the following lines and report this to support@ttcontrol.com ');
      | disp('<< begin of error message dump >>');
      | disp(['Version of TTC580-BlockLib: ', get_param(gcb,'tt_iolib_version')]);
      | disp(get_param(gcb,'ttDescription'));
      | disp(gcb);
      | x=lasterror;disp(x.message);
      | disp(get_param(gcb,'MaskValues'));
      | disp(version);
      | disp(computer);
      | disp('<< end of error message dump >>');
      | disp('------------------------------------------------------------');
      | disp(' ');
      | %Standard catch section END
      | end
      mask help: Write data to serial interface.
      mask init:
      | %
      settings: CopyFcn=%deleted  RTWSystemCode=Inline
      mask Help: No further help available for this block
  Logical Operator : Logic  AllPortsSameDT=off  OutDataTypeStr=boolean
  Saturation Dynamic : simulink/Discontinuities/Saturation Dynamic  OutMin=[]  OutMax=[]  OutDataTypeStr=uint16  OutputDataTypeScalingMode=uint16  OutDataType=fixdt(1, 16)  OutScaling=2^-10  DoSatur=off
  Terminator2 : Terminator
  Terminator_value1 : Terminator
  Terminator_value2 : Terminator
  Trigger : Subsystem  mask(Derate Trigger){derate=derate_val}
      mask help: derate "n": every n-th cylce a trigger is submitted
  Width : Width  DataType=uint16
  snprintf_merge_printf : Subsystem  LoadFcn=|  mask(snprintf_merge_printf_Code){SampleTime=-1, ttlib=IO_Blk_Lib_TTC500, ttDescription=snprintf_merge_printf, tt_iolib_version=0.25, max_size=80, Comment=['\033[0;32m',Comment,'\033[0m']}
      | try
      | %
      | %Upgrade Information - standard BEGIN
      | new_color = 'blue';
      | new_ver = '0.25';
      | act_ver = get_param(gcb,'tt_iolib_version');
      | if not(strcmp(act_ver,new_ver))
      |     disp(['Upgrade block: ',gcb,char(10),'       Version: ',act_ver,' to ',new_ver]);
      |     %switch - case for specific upgrade information e.g. additional parameter required 
      |     %Change appearance and version information
      |     set_param(gcb,'ForegroundColor',new_color);
      |     set_param(gcb,'tt_iolib_version',new_ver);
      | end
      | %Upgrade Information - standard END
      | catch
      | %Standard catch section BEGIN
      | errordlg('An error occurred in a callback of the TTC580-BlockLib. Please open the Diagnostic Viewer for further details');
      | disp(' ');
      | disp('------------------------------------------------------------');
      | disp('An error occurred in a callback of the TTC580-BlockLib.');
      | disp(['Please check the parameters in the mask of ',gcb]);
      | disp('If you do not encounter any violations, then please '); 
      | disp('copy the following lines and report this to support@ttcontrol.com ');
      | disp('<< begin of error message dump >>');
      | disp(['Version of TTC580-BlockLib: ', get_param(gcb,'tt_iolib_version')]);
      | disp(get_param(gcb,'ttDescription'));
      | disp(gcb);
      | x=lasterror;disp(x.message);
      | disp(get_param(gcb,'MaskValues'));
      | disp(version);
      | disp(computer);
      | disp('<< end of error message dump >>');
      | disp('------------------------------------------------------------');
      | disp(' ');
      | %Standard catch section END
      | end
      mask help:
      | The C library function snprintf sends formatted output to a string with maximum length of n characters.
      | This snprintf implementation adds LF and reset cursor information the way that the printf implementation did it before
      mask init:
      | %
      settings: CopyFcn=%deleted
      mask Help: No further help available for this block
      mask Callback max_size: %
      mask Callback Comment: %
  wires:
  Data Type Conversion/1 -> Saturation Dynamic/2
  IO_UART_Write/1(ErrorCode) -> Terminator_value1/1
  Constant/1 -> Saturation Dynamic/3
  value/1 -> snprintf_merge_printf/1(value), Compare To Zero/1
  snprintf_merge_printf/1(NumOfChar) -> Data Type Conversion/1
  Width/1 -> Saturation Dynamic/1
  IO_UART_Init/1(ErrorCode) -> Terminator_value2/1
  Saturation Dynamic/1 -> IO_UART_Write/2(len)
  snprintf_merge_printf/2(str_out) -> IO_UART_Write/1(data), Width/1
  IO_UART_Write/2(tx_len) -> Terminator2/1
  Trigger/1(Trigger) -> Logical Operator/1
  Compare To Zero/1 -> Logical Operator/2
  Logical Operator/1 -> IO_UART_Write/Enable
